simulink model "mpc_tmp"
settings: Solver=ode45  StartTime=0.0  StopTime=1000  RelTol=1e-3
PreLoadFcn:
  | load mpc_tmpdemodata;
  | mpctmpinit
values from neighbouring files (symbols this model uses):
  Fb0 = 3.55555555556    [mpc_tmpdata.mat]
  Fbh0 = 6.82828282828    [mpc_tmpdata.mat]
  ke = 12.7272727273    [mpc_tmpdata.mat]
  ke2 = 12.2245913291    [mpc_tmpdata.mat]
  kf = 0.20751953125    [mpc_tmpdata.mat]
  kf2 = 0.170918367347    [mpc_tmpdata.mat]
  m2 = 106.666666667    [mpc_tmpdata.mat]
  M2 = 266.666666667    [mpc_tmpdata.mat]
  SAMPLING_INTERVAL = 10    [main_code.m]    (also in main_using_Torsche.m)
  x_new_product_setpoint = task{subtask_num}.set_point    [main_code.m]    (also in main_using_Torsche.m = task(subtask_num).set_point)
  x_product_id = task{subtask_num}.product_id    [main_code.m]    (also in main_using_Torsche.m = task(subtask_num).product_id)
libraries: cstblocks x9, simulink x4, mpclib x1
settings Model: FPTRunName=Active  Creator=jowen  LastModifiedBy=manoj
settings DataIOCC: LimitDataPoints=on  SaveFinalState=on  SaveFormat=Array  SignalLoggingSaveFormat=ModelDataLogs  ReturnWorkspaceOutputs=off  SignalLoggingName=logsOut
settings OptimizationCC: ExpressionDepthLimit=2147483647  InitFltsAndDblsToZero=on  LifeSpan=inf  SimCompilerOptimization=Off
settings DebuggingCC: SaveWithParameterizedLinksMsg=none  UnderspecifiedInitializationDetection=Classic  MergeDetectMultiDrivingBlocksExec=none  CheckExecutionContextPreStartOutputMsg=on  CheckExecutionContextRuntimeOutputMsg=on  SignalResolutionControl=TryResolveAllWithWarning  MultiTaskDSMMsg=warning  MultiTaskCondExecSysMsg=none  FcnCallInpInsideContextMsg=Enable All  FrameProcessingCompatibilityMsg=warning  StateNameClashWarn=warning  StrictBusMsg=None  SFUnexpectedBacktrackingDiag=warning  SFNoUnconditionalDefaultTransitionDiag=warning
settings HardwareCC: ProdBitPerPointer=32  ProdLargestAtomicFloat=None  ProdIntDivRoundTo=Undefined  ProdEndianess=Unspecified  ProdWordSize=32  ProdHWDeviceType=32-bit Generic
settings ModelReferenceCC: PropagateSignalLabelsOutOfModel=off
settings SFSimCC: SimUseLocalCustomCode=off
settings RTWCC: RTWUseLocalCustomCode=off  IncludeERTFirstTime=on  RTWCompilerOptimization=Off
settings GRTTargetCC: TargetFcnLib=ansi_tfl_tmw.mat  CodeReplacementLibrary=ANSI_C  GeneratePreprocessorConditionals=Disable all  CombineOutputUpdateFcns=off  CPPClassGenCompliant=off  GRTInterface=on

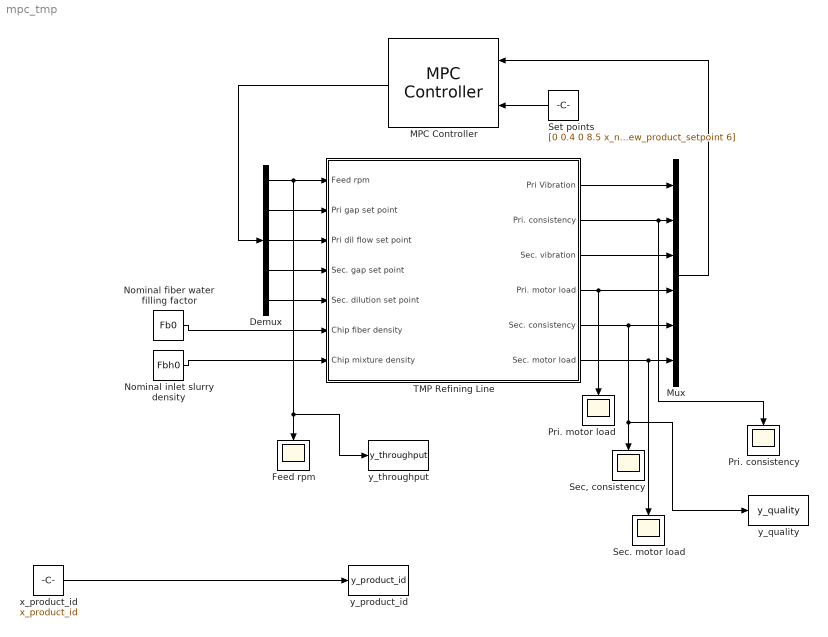
== system mpc_tmp ==
  Demux : Demux  Outputs=5
  Feed rpm : Scope
      settings: YMin=0.3825  YMax=0.415  SaveName=ScopeData4
  MPC Controller : mpclib/MPC Controller  mpcobj=MPC1  x0=[]  md_inport=off  mv_inport=off  lims_inport=off  switch_inport=off  ywt_inport=off  duwt_inport=off  rhoeps_inport=off  cost_outport=off  return_sequence=off  return_qpstatus=off  is_multiple=0  enable_value=0  n_mv=5  n_mo=6  n_md=0  n_ts=0.5  is_designfromscratch=0  ref_from_ws=off  ref_signal_name=[]  ref_preview=on  md_from_ws=off  md_signal_name=[]  md_preview=on  from_project=off  project_file=MPCtask.mat
  Mux : Mux  Inputs=6
  Nominal fiber water filling factor : Constant  Value=Fb0
  Nominal inlet slurry density : Constant  Value=Fbh0
  Pri. consistency : Scope
      settings: YMin=0.3825  YMax=0.415  SaveName=ScopeData3
  Pri. motor load : Scope
      settings: YMin=0.3825  YMax=0.415
  "Sec, consistency" : Scope
      settings: YMin=0.3825  YMax=0.415
  Sec. motor load : Scope
      settings: YMin=0.3825  YMax=0.415  SaveName=ScopeData2
  Set points : Constant  Value=[0 0.4 0 8.5 x_new_product_setpoint 6]  VectorParams1D=off
  TMP Refining Line : Subsystem
  x_product_id : Constant  Value=x_product_id
  y_product_id : ToWorkspace  VariableName=y_product_id  SampleTime=SAMPLING_INTERVAL  SaveFormat=Timeseries
  y_quality : ToWorkspace  VariableName=y_quality  SampleTime=SAMPLING_INTERVAL  SaveFormat=Timeseries
  y_throughput : ToWorkspace  VariableName=y_throughput  SampleTime=SAMPLING_INTERVAL  SaveFormat=Timeseries
  wires:
  Demux/1 -> y_throughput/1, Feed rpm/1, TMP Refining Line/1(Feed rpm)
  Demux/3 -> TMP Refining Line/3(Pri dil flow set point)
  Demux/4 -> TMP Refining Line/4(Sec. gap set point)
  Demux/5 -> TMP Refining Line/5(Sec. dilution set point)
  TMP Refining Line/1(Pri Vibration) -> Mux/1
  TMP Refining Line/2(Pri. consistency) -> Pri. consistency/1, Mux/2
  TMP Refining Line/3(Sec. vibration) -> Mux/3
  TMP Refining Line/4(Pri. motor load) -> Mux/4, Pri. motor load/1
  TMP Refining Line/5(Sec. consistency) -> Mux/5, y_quality/1, "Sec, consistency"/1
  TMP Refining Line/6(Sec. motor load) -> Mux/6, Sec. motor load/1
  Mux/1 -> MPC Controller/1
  Set points/1 -> MPC Controller/2
  Demux/2 -> TMP Refining Line/2(Pri gap set point)
  Nominal fiber water filling factor/1 -> TMP Refining Line/6(Chip fiber density)
  MPC Controller/1 -> Demux/1
  Nominal inlet slurry density/1 -> TMP Refining Line/7(Chip mixture density)
  x_product_id/1 -> y_product_id/1

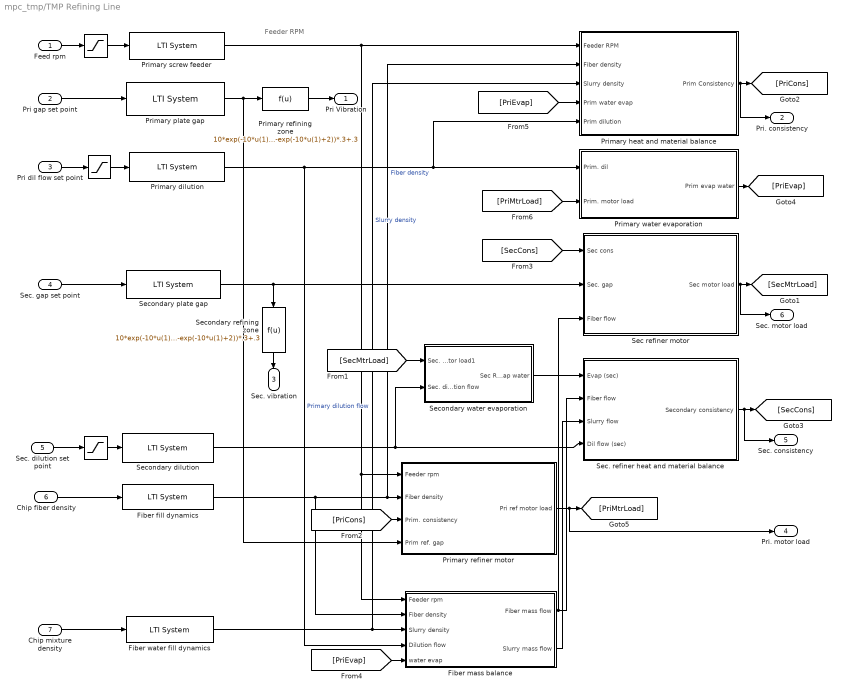
== system mpc_tmp/TMP Refining Line ==
  note: Feeder RPM
  Feed rpm : Inport
  Pri gap set point : Inport  Port=2
  Pri dil flow set point : Inport  Port=3
  Sec. gap set point : Inport  Port=4
  Sec. dilution set point : Inport  Port=5
  Chip fiber density : Inport  Port=6
  Chip mixture density : Inport  Port=7
  "  " : Saturate  UpperLimit=35  LowerLimit=25  SampleTime=0.5
  "    " : Saturate  UpperLimit=200  LowerLimit=90  SampleTime=0.5
  "       " : Saturate  UpperLimit=200  LowerLimit=90  SampleTime=0.5
  Fiber fill dynamics : cstblocks/LTI System  sys=FiberFill  IC=Fb0
  Fiber mass balance : Subsystem
  Fiber water fill dynamics : cstblocks/LTI System  sys=FiberWaterFill  IC=Fbh0
  Primary dilution : cstblocks/LTI System  sys=DilFlowPrimary  IC=dp0
  Primary heat and material balance : Subsystem
  Primary plate gap : cstblocks/LTI System  sys=PlateGapPrimary  IC=gp0
  Primary refiner motor : Subsystem
  Primary refining zone : Fcn  Expr=10*exp(-10*u(1)+2)*(1.26-0.3*u(1))-(1-exp(-10*u(1)+2))*.3+.3
  Primary screw feeder : cstblocks/LTI System  sys=ChipFeeder  IC=vp0
  Primary water evaporation : Subsystem
  Sec refiner motor : Subsystem
  Sec. refiner heat and material balance : Subsystem
  "Secondary dilution " : cstblocks/LTI System  sys=DilFlowSecondary  IC=gs0
  Secondary plate gap : cstblocks/LTI System  sys=PlateGapSecondary  IC=gs0
  Secondary refining zone : Fcn  Expr=10*exp(-10*u(1)+2)*(1.26-0.3*u(1))-(1-exp(-10*u(1)+2))*.3+.3  SampleTime=0.5
  Secondary water evaporation : Subsystem
  Pri Vibration : Outport
  Pri. consistency : Outport  Port=2
  Sec. vibration : Outport  Port=3
  Pri. motor load : Outport  Port=4
  Sec. consistency : Outport  Port=5
  Sec. motor load : Outport  Port=6
  wires:
  "  "/1 -> Primary screw feeder/1
  Primary plate gap/1 -> Primary refining zone/1, Primary refiner motor/4(Prim ref. gap)
  Secondary plate gap/1 -> Secondary refining zone/1, Sec refiner motor/2(Sec. gap)
  "    "/1 -> Primary dilution/1
  "       "/1 -> "Secondary dilution "/1
  "Secondary dilution "/1 -> Sec. refiner heat and material balance/4(Dil flow (sec)), Secondary water evaporation/2(Sec. dilution flow)
  Sec. dilution set point/1 -> "       "/1
  Fiber water fill dynamics/1 -> Primary heat and material balance/3(Slurry density), Fiber mass balance/3(Slurry density)  "Slurry density"
  Fiber fill dynamics/1 -> Fiber mass balance/2(Fiber density), Primary heat and material balance/2(Fiber density), Primary refiner motor/2(Fiber density)  "Fiber density"
  Primary dilution/1 -> Primary water evaporation/1(Prim. dil), Primary heat and material balance/5(Prim dilution), Fiber mass balance/4(Dilution flow)  "Primary dilution flow"
  Primary screw feeder/1 -> Primary heat and material balance/1(Feeder RPM), Fiber mass balance/1(Feeder rpm), Primary refiner motor/1(Feeder rpm)
  Fiber mass balance/1(Fiber mass flow) -> Sec. refiner heat and material balance/2(Fiber flow), Sec refiner motor/3(Fiber flow)
  Fiber mass balance/2(Slurry mass flow) -> Sec. refiner heat and material balance/3(Slurry flow)
  Secondary water evaporation/1(Sec Ref. evap water) -> Sec. refiner heat and material balance/1(Evap (sec))
  Primary refining zone/1 -> Pri Vibration/1
  Sec refiner motor/1(Sec motor load) -> [SecMtrLoad], Sec. motor load/1
  Primary heat and material balance/1(Prim Consistency) -> [PriCons], Pri. consistency/1
  [PriCons] -> Primary refiner motor/3(Prim. consistency)
  Sec. refiner heat and material balance/1(Secondary consistency) -> [SecCons], Sec. consistency/1
  [SecCons] -> Sec refiner motor/1(Sec cons)
  Primary water evaporation/1(Prim evap water) -> [PriEvap]
  [PriEvap] -> Primary heat and material balance/4(Prim water evap)
  Primary refiner motor/1(Pri ref motor load) -> [PriMtrLoad], Pri. motor load/1
  [PriMtrLoad] -> Primary water evaporation/2(Prim. motor load)
  [SecMtrLoad] -> Secondary water evaporation/1(Sec. motor load1)
  Feed rpm/1 -> "  "/1
  Pri gap set point/1 -> Primary plate gap/1
  Pri dil flow set point/1 -> "    "/1
  Sec. gap set point/1 -> Secondary plate gap/1
  Secondary refining zone/1 -> Sec. vibration/1
  [PriEvap] -> Fiber mass balance/5(water evap)
  Chip fiber density/1 -> Fiber fill dynamics/1
  Chip mixture density/1 -> Fiber water fill dynamics/1

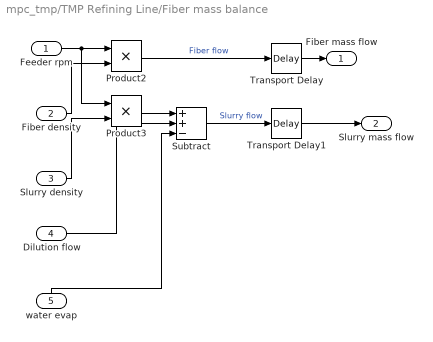
== system mpc_tmp/TMP Refining Line/Fiber mass balance ==
  Feeder rpm : Inport
  Fiber density : Inport  Port=2
  Slurry density : Inport  Port=3
  Dilution flow : Inport  Port=4
  water evap : Inport  Port=5
  Product2 : Product  RndMeth=Zero
  Product3 : Product  RndMeth=Zero
  Subtract : Sum  Inputs=++-
  Transport Delay : TransportDelay  DelayTime=2  InitialOutput=m2
  Transport Delay1 : TransportDelay  DelayTime=2  InitialOutput=M2
  Fiber mass flow : Outport
  Slurry mass flow : Outport  Port=2
  wires:
  Product2/1 -> Transport Delay/1  "Fiber flow"
  Product3/1 -> Subtract/1
  Subtract/1 -> Transport Delay1/1  "Slurry flow"
  Feeder rpm/1 -> Product2/1, Product3/1
  Fiber density/1 -> Product2/2
  Slurry density/1 -> Product3/2
  Dilution flow/1 -> Subtract/2
  water evap/1 -> Subtract/3
  Transport Delay/1 -> Fiber mass flow/1
  Transport Delay1/1 -> Slurry mass flow/1

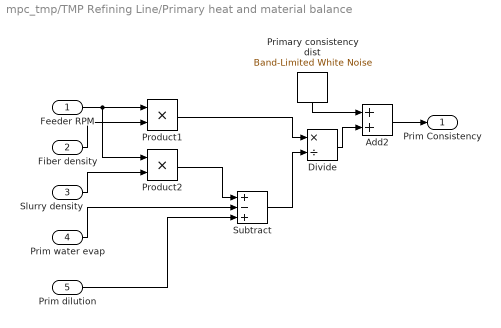
== system mpc_tmp/TMP Refining Line/Primary heat and material balance ==
  Feeder RPM : Inport
  Fiber density : Inport  Port=2
  Slurry density : Inport  Port=3
  Prim water evap : Inport  Port=4
  Prim dilution : Inport  Port=5
  Add2 : Sum
  Divide : Product  Inputs=*/  SampleTime=.5
  Primary consistency dist : simulink/Sources/Band-Limited White Noise  Cov=0.00001  Ts=0.5  seed=[23341]
  Product1 : Product  RndMeth=Zero
  Product2 : Product  RndMeth=Zero
  Subtract : Sum  Inputs=+-+
  Prim Consistency : Outport
  wires:
  Product2/1 -> Subtract/1
  Subtract/1 -> Divide/2
  Product1/1 -> Divide/1
  Divide/1 -> Add2/2
  Primary consistency dist/1 -> Add2/1
  Feeder RPM/1 -> Product1/1, Product2/1
  Prim dilution/1 -> Subtract/3
  Add2/1 -> Prim Consistency/1
  Fiber density/1 -> Product1/2
  Slurry density/1 -> Product2/2
  Prim water evap/1 -> Subtract/2

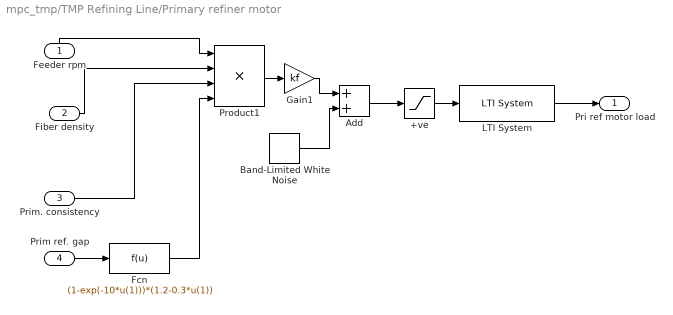
== system mpc_tmp/TMP Refining Line/Primary refiner motor ==
  Feeder rpm : Inport
  Fiber density : Inport  Port=2
  Prim. consistency : Inport  Port=3
  Prim ref. gap : Inport  Port=4
  +ve : Saturate  UpperLimit=inf  LowerLimit=0  SampleTime=0.5
  Add : Sum
  Band-Limited White Noise : simulink/Sources/Band-Limited White Noise  Cov=0.0001  Ts=0.5  seed=[23341]
  Fcn : Fcn  Expr=(1-exp(-10*u(1)))*(1.2-0.3*u(1))
  Gain1 : Gain  Gain=kf
  LTI System : cstblocks/LTI System  sys=UnitDelay  IC=mlp0
  Product1 : Product  Inputs=4  RndMeth=Zero
  Pri ref motor load : Outport
  wires:
  Product1/1 -> Gain1/1
  Fcn/1 -> Product1/4
  Gain1/1 -> Add/1
  Add/1 -> +ve/1
  Band-Limited White Noise/1 -> Add/2
  Feeder rpm/1 -> Product1/1
  Fiber density/1 -> Product1/2
  Prim ref. gap/1 -> Fcn/1
  Prim. consistency/1 -> Product1/3
  +ve/1 -> LTI System/1
  LTI System/1 -> Pri ref motor load/1

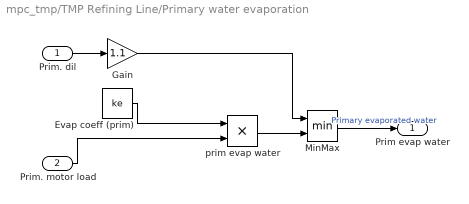
== system mpc_tmp/TMP Refining Line/Primary water evaporation ==
  Prim. dil : Inport
  Prim. motor load : Inport  Port=2
  Evap coeff (prim) : Constant  Value=ke
  Gain : Gain  Gain=1.1
  MinMax : MinMax  Inputs=2
  prim evap water : Product  RndMeth=Zero
  Prim evap water : Outport
  wires:
  Evap coeff (prim)/1 -> prim evap water/1
  prim evap water/1 -> MinMax/2
  Gain/1 -> MinMax/1
  Prim. dil/1 -> Gain/1
  MinMax/1 -> Prim evap water/1  "Primary evaporated water"
  Prim. motor load/1 -> prim evap water/2

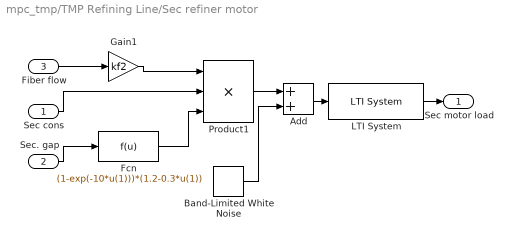
== system mpc_tmp/TMP Refining Line/Sec refiner motor ==
  Sec cons : Inport
  Sec. gap : Inport  Port=2
  Fiber flow : Inport  Port=3
  Add : Sum
  Band-Limited White Noise : simulink/Sources/Band-Limited White Noise  Cov=0.0001  Ts=0.5  seed=[23341]
  Fcn : Fcn  Expr=(1-exp(-10*u(1)))*(1.2-0.3*u(1))
  Gain1 : Gain  Gain=kf2
  LTI System : cstblocks/LTI System  sys=UnitDelay  IC=mls0
  Product1 : Product  Inputs=3  RndMeth=Zero
  Sec motor load : Outport
  wires:
  Gain1/1 -> Product1/1
  Fcn/1 -> Product1/3
  Product1/1 -> Add/1
  Band-Limited White Noise/1 -> Add/2
  Fiber flow/1 -> Gain1/1
  Sec. gap/1 -> Fcn/1
  Sec cons/1 -> Product1/2
  Add/1 -> LTI System/1
  LTI System/1 -> Sec motor load/1

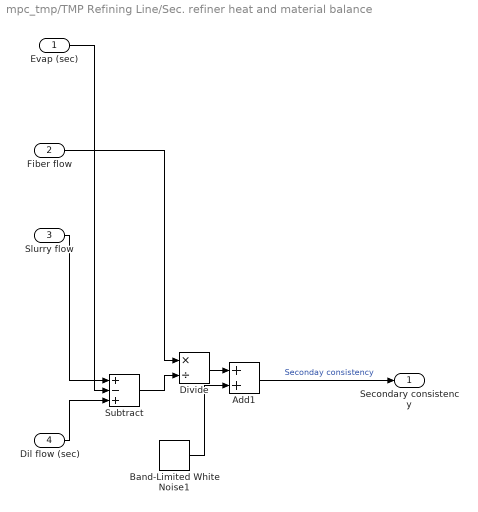
== system mpc_tmp/TMP Refining Line/Sec. refiner heat and material balance ==
  Evap (sec) : Inport
  Fiber flow : Inport  Port=2
  Slurry flow : Inport  Port=3
  Dil flow (sec) : Inport  Port=4
  Add1 : Sum
  Band-Limited White Noise1 : simulink/Sources/Band-Limited White Noise  Cov=0.00001  Ts=0.5  seed=[23341]
  Divide : Product  Inputs=*/  SampleTime=.5
  Subtract : Sum  Inputs=+-+
  Secondary consistency : Outport
  wires:
  Evap (sec)/1 -> Subtract/2
  Subtract/1 -> Divide/2
  Divide/1 -> Add1/1
  Band-Limited White Noise1/1 -> Add1/2
  Fiber flow/1 -> Divide/1
  Dil flow (sec)/1 -> Subtract/3
  Add1/1 -> Secondary consistency/1  "Seconday consistency"
  Slurry flow/1 -> Subtract/1

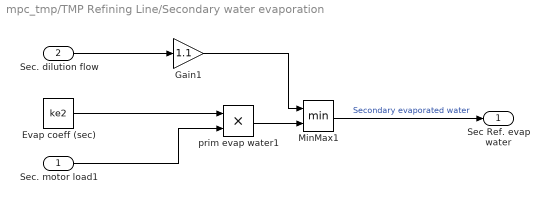
== system mpc_tmp/TMP Refining Line/Secondary water evaporation ==
  Sec. motor load1 : Inport
  Sec. dilution flow : Inport  Port=2
  Evap coeff (sec) : Constant  Value=ke2
  Gain1 : Gain  Gain=1.1
  MinMax1 : MinMax  Inputs=2
  prim evap water1 : Product  RndMeth=Zero
  Sec Ref. evap water : Outport
  wires:
  Evap coeff (sec)/1 -> prim evap water1/1
  prim evap water1/1 -> MinMax1/2
  Sec. dilution flow/1 -> Gain1/1
  Sec. motor load1/1 -> prim evap water1/2
  Gain1/1 -> MinMax1/1
  MinMax1/1 -> Sec Ref. evap water/1  "Secondary evaporated water"
